simulink model "madgwick_bias"  (R2016a)
settings: Solver=VariableStepAuto  StartTime=0.0  StopTime=10.0  RelTol=1e-3
settings Model: Creator=mgreiff  LastModifiedBy=mgreiff
settings DataIOCC: LimitDataPoints=on
settings DebuggingCC: AllowSymbolicDim=off
settings ModelReferenceCC: PropagateSignalLabelsOutOfModel=off
settings GRTTargetCC: GeneratePreprocessorConditionals=Use local settings

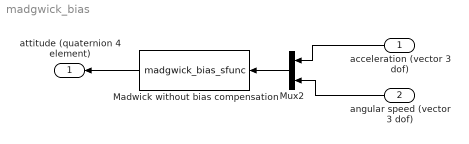
== system madgwick_bias ==
  acceleration (vector 3 dof) : Inport  PortDimensions=3
  angular speed (vector 3 dof) : Inport  Port=2  PortDimensions=3
  Madwick without bias compensation : S-Function  FunctionName=madgwick_bias_sfunc  Parameters=MADparam  SFunctionDeploymentMode=off  EnableBusSupport=off
  Mux2 : Mux  Inputs=2
  attitude (quaternion 4 element) : Outport
  wires:
  acceleration (vector 3 dof)/1 -> Mux2/1
  angular speed (vector 3 dof)/1 -> Mux2/2
  Madwick without bias compensation/1 -> attitude (quaternion 4 element)/1
  Mux2/1 -> Madwick without bias compensation/1
